simulink model "linearaircraft"  (R2023a)
settings: Solver=VariableStepAuto  StartTime=0.0  StopTime=15  MaxStep=1e-3  RelTol=1e-3
undefined symbols (not defined in the file or in its folder): latdyn, londyn
settings Model: Creator=ebube  LastModifiedBy=ebube

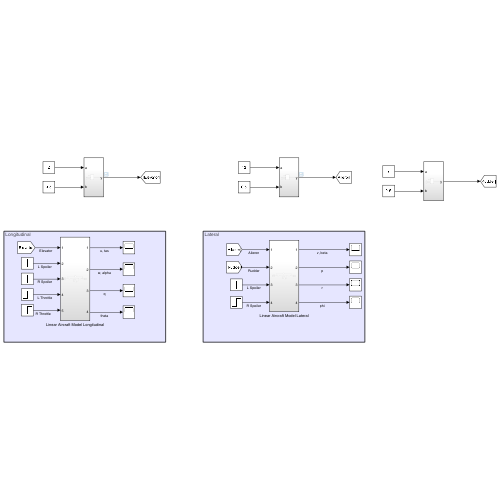
[thumbnail: Simulink's stored preview of the top-level diagram]
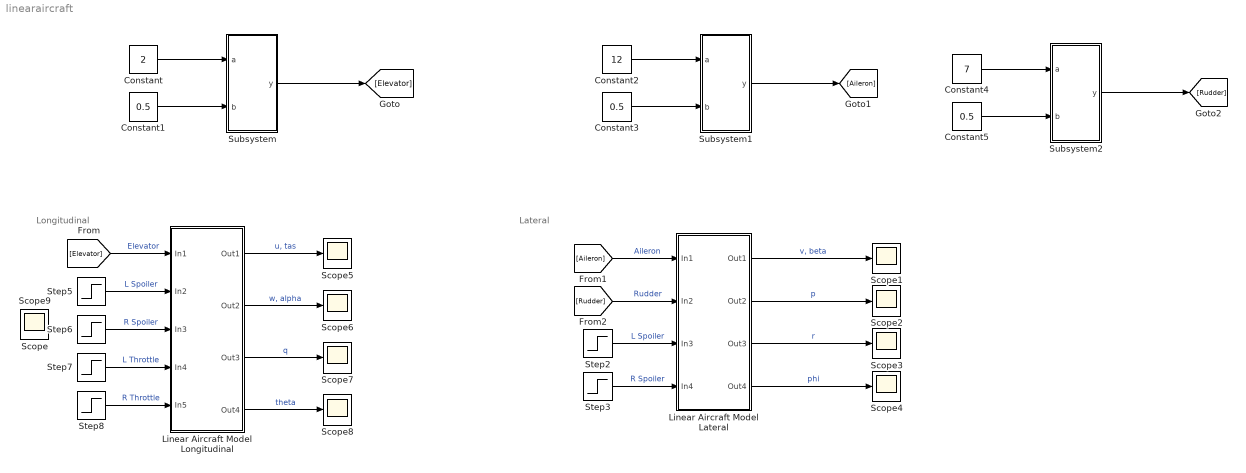
== system linearaircraft ==
  note: Longitudinal
  note: Lateral
  Constant : Constant  Value=2
  Constant1 : Constant  Value=0.5
  Constant2 : Constant  Value=12
  Constant3 : Constant  Value=0.5
  Constant4 : Constant  Value=7
  Constant5 : Constant  Value=0.5
  Linear Aircraft Model Lateral : Subsystem
  Linear Aircraft Model Longitudinal : Subsystem
  Scope{,1..9} (10 alike) : Scope
  Step{2..3,5..8} (6 alike) : Step  After=0  SampleTime=0
  Subsystem : Subsystem
  Subsystem1 : Subsystem
  Subsystem2 : Subsystem
  wires:
  [Aileron] -> Linear Aircraft Model Lateral/1(In1)  "Aileron"
  Linear Aircraft Model Lateral/1(Out1) -> Scope1/1  "v, beta"
  [Rudder] -> Linear Aircraft Model Lateral/2(In2)  "Rudder"
  Linear Aircraft Model Lateral/2(Out2) -> Scope2/1  "p"
  Linear Aircraft Model Lateral/3(Out3) -> Scope3/1  "r"
  Linear Aircraft Model Lateral/4(Out4) -> Scope4/1  "phi"
  Step2/1 -> Linear Aircraft Model Lateral/3(In3)  "L Spoiler"
  Step3/1 -> Linear Aircraft Model Lateral/4(In4)  "R Spoiler"
  Step7/1 -> Linear Aircraft Model Longitudinal/4(In4)  "L Throttle"
  Step6/1 -> Linear Aircraft Model Longitudinal/3(In3)  "R Spoiler"
  Linear Aircraft Model Longitudinal/4(Out4) -> Scope8/1  "theta"
  Linear Aircraft Model Longitudinal/3(Out3) -> Scope7/1  "q"
  Linear Aircraft Model Longitudinal/2(Out2) -> Scope6/1  "w, alpha"
  Step5/1 -> Linear Aircraft Model Longitudinal/2(In2)  "L Spoiler"
  Linear Aircraft Model Longitudinal/1(Out1) -> Scope5/1  "u, tas"
  [Elevator] -> Linear Aircraft Model Longitudinal/1(In1)  "Elevator"
  Step8/1 -> Linear Aircraft Model Longitudinal/5(In5)  "R Throttle"
  Constant/1 -> Subsystem/1(a)
  Subsystem/1(y) -> [Elevator]
  Constant1/1 -> Subsystem/2(b)
  Subsystem1/1(y) -> [Aileron]
  Constant2/1 -> Subsystem1/1(a)
  Constant3/1 -> Subsystem1/2(b)
  Constant5/1 -> Subsystem2/2(b)
  Constant4/1 -> Subsystem2/1(a)
  Subsystem2/1(y) -> [Rudder]

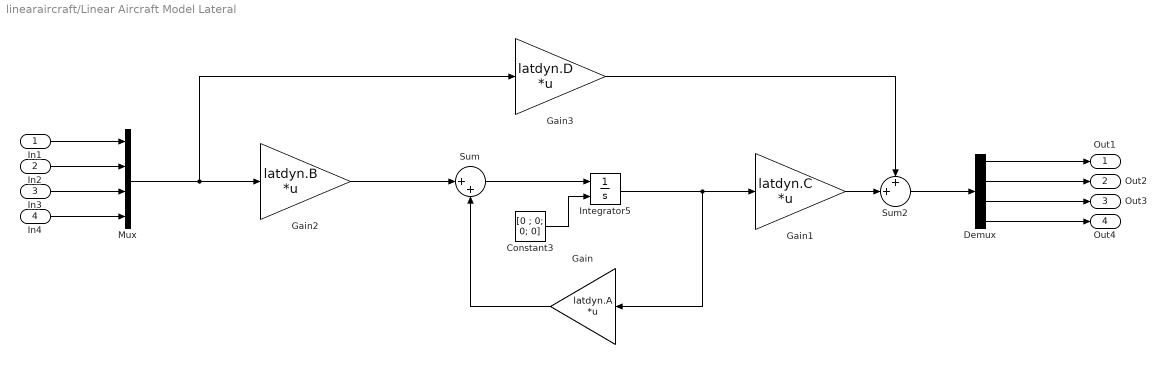
== system linearaircraft/Linear Aircraft Model Lateral ==
  In1 : Inport
  In2 : Inport  Port=2
  In3 : Inport  Port=3
  In4 : Inport  Port=4
  Constant3 : Constant  Value=[0 ; 0; 0; 0]  VectorParams1D=off
  Demux : Demux
  Gain : Gain  Gain=latdyn.A  Multiplication=Matrix(K*u)
  Gain1 : Gain  Gain=latdyn.C  Multiplication=Matrix(K*u)
  Gain2 : Gain  Gain=latdyn.B  Multiplication=Matrix(K*u)
  Gain3 : Gain  Gain=latdyn.D  Multiplication=Matrix(K*u)
  Integrator5 : Integrator  InitialConditionSource=external
  Mux : Mux
  Sum : Sum  Inputs=|++
  Sum2 : Sum  Inputs=++|
  Out1 : Outport
  Out2 : Outport  Port=2
  Out3 : Outport  Port=3
  Out4 : Outport  Port=4
  wires:
  Constant3/1 -> Integrator5/2
  Gain2/1 -> Sum/1
  Gain/1 -> Sum/2
  Sum/1 -> Integrator5/1
  Demux/1 -> Out1/1
  Demux/2 -> Out2/1
  Demux/3 -> Out3/1
  Demux/4 -> Out4/1
  Integrator5/1 -> Gain1/1, Gain/1
  Gain3/1 -> Sum2/1
  Mux/1 -> Gain3/1, Gain2/1
  In1/1 -> Mux/1
  In2/1 -> Mux/2
  In3/1 -> Mux/3
  In4/1 -> Mux/4
  Gain1/1 -> Sum2/2
  Sum2/1 -> Demux/1

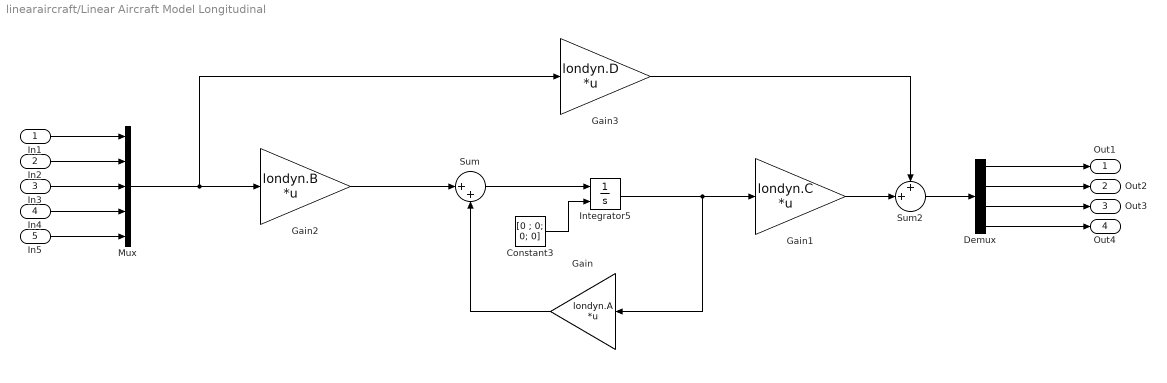
== system linearaircraft/Linear Aircraft Model Longitudinal ==
  In1 : Inport
  In2 : Inport  Port=2
  In3 : Inport  Port=3
  In4 : Inport  Port=4
  In5 : Inport  Port=5
  Constant3 : Constant  Value=[0 ; 0; 0; 0]  VectorParams1D=off
  Demux : Demux
  Gain : Gain  Gain=londyn.A  Multiplication=Matrix(K*u)
  Gain1 : Gain  Gain=londyn.C  Multiplication=Matrix(K*u)
  Gain2 : Gain  Gain=londyn.B  Multiplication=Matrix(K*u)
  Gain3 : Gain  Gain=londyn.D  Multiplication=Matrix(K*u)
  Integrator5 : Integrator  InitialConditionSource=external
  Mux : Mux  Inputs=5
  Sum : Sum  Inputs=|++
  Sum2 : Sum  Inputs=++|
  Out1 : Outport
  Out2 : Outport  Port=2
  Out3 : Outport  Port=3
  Out4 : Outport  Port=4
  wires:
  In4/1 -> Mux/4
  In3/1 -> Mux/3
  In2/1 -> Mux/2
  In1/1 -> Mux/1
  Mux/1 -> Gain2/1, Gain3/1
  Demux/4 -> Out4/1
  Demux/3 -> Out3/1
  Demux/2 -> Out2/1
  Demux/1 -> Out1/1
  Sum/1 -> Integrator5/1
  Gain/1 -> Sum/2
  Gain2/1 -> Sum/1
  Constant3/1 -> Integrator5/2
  Integrator5/1 -> Gain1/1, Gain/1
  In5/1 -> Mux/5
  Sum2/1 -> Demux/1
  Gain1/1 -> Sum2/2
  Gain3/1 -> Sum2/1

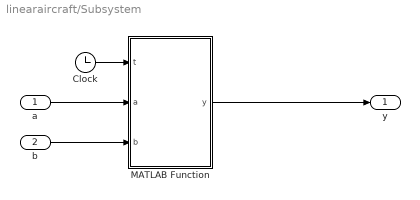
== system linearaircraft/Subsystem ==
  a : Inport
  b : Inport  Port=2
  Clock : Clock
  MATLAB Function : MATLAB Function  TreatAsAtomicUnit=on
  y : Outport
  wires:
  b/1 -> MATLAB Function/3(b)
  a/1 -> MATLAB Function/2(a)
  MATLAB Function/1(y) -> y/1
  Clock/1 -> MATLAB Function/1(t)

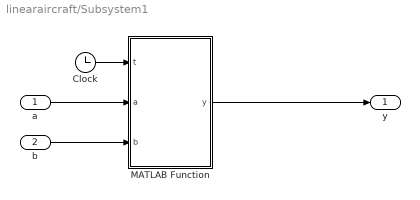
== system linearaircraft/Subsystem1 ==
  a : Inport
  b : Inport  Port=2
  Clock : Clock
  MATLAB Function : MATLAB Function  TreatAsAtomicUnit=on
  y : Outport
  wires:
  b/1 -> MATLAB Function/3(b)
  a/1 -> MATLAB Function/2(a)
  MATLAB Function/1(y) -> y/1
  Clock/1 -> MATLAB Function/1(t)

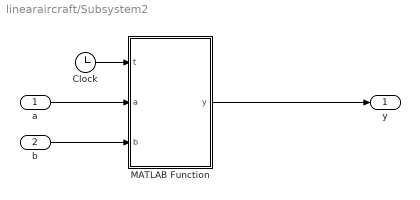
== system linearaircraft/Subsystem2 ==
  a : Inport
  b : Inport  Port=2
  Clock : Clock
  MATLAB Function : MATLAB Function  TreatAsAtomicUnit=on
  y : Outport
  wires:
  Clock/1 -> MATLAB Function/1(t)
  MATLAB Function/1(y) -> y/1
  a/1 -> MATLAB Function/2(a)
  b/1 -> MATLAB Function/3(b)

== matlab function linearaircraft/Subsystem/MATLAB Function ==
  data: t input; y output; a input; b input
function y = fcn(t, a, b)
    if t>a && t<a+b
        y = 1;
    elseif t>a+b && t<a+2*b
        y = -1;
    else
        y = 0;
    end
end

== matlab function linearaircraft/Subsystem2/MATLAB Function ==
  data: t input; y output; a input; b input
function y = fcn(t, a, b)
    if t>a && t<a+b
        y = 1;
    elseif t>a+b && t<a+2*b
        y = -1;
    else
        y = 0;
    end
end

== matlab function linearaircraft/Subsystem1/MATLAB Function ==
  data: t input; y output; a input; b input
function y = fcn(t, a, b)
    if t>a && t<a+b
        y = 1;
    elseif t>a+b && t<a+2*b
        y = -1;
    else
        y = 0;
    end
end
